simulink subsystem "Trot_planning"  (R2022b)
settings: Solver=VariableStepAuto  StartTime=0.0  StopTime=10.0  RelTol=1e-3
undefined symbols (not defined in the file or in its folder): D, DiscIntNeverNeededParam, P
settings Model: Creator=LiAn  LastModifiedBy=LiAn

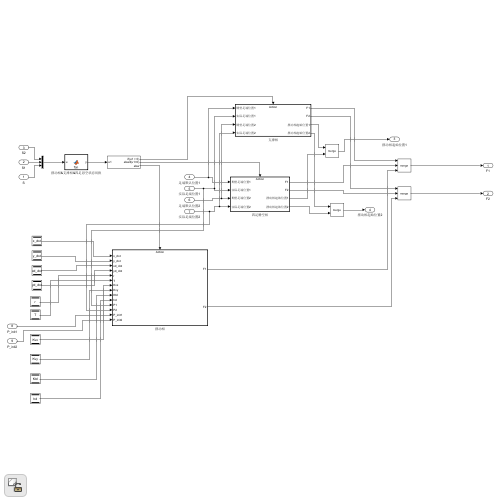
[thumbnail: Simulink's stored preview of the top-level diagram]
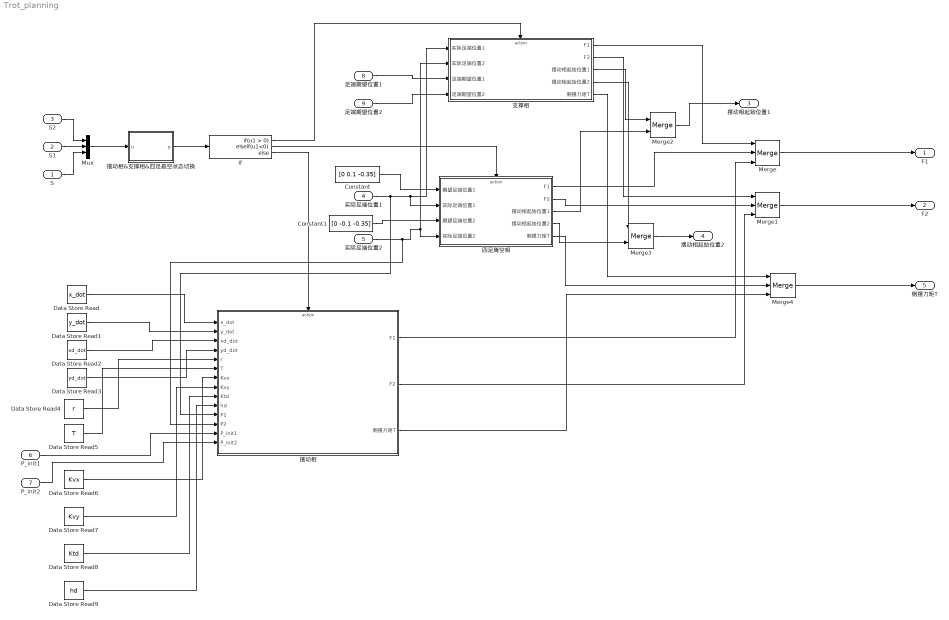
== system Trot_planning ==
  S : Inport
  S1 : Inport  Port=2
  S2 : Inport  Port=3
  实际足端位置1 : Inport  Port=4
  实际足端位置2 : Inport  Port=5
  P_init1 : Inport  Port=6
  P_init2 : Inport  Port=7
  足端期望位置1 : Inport  Port=8
  足端期望位置2 : Inport  Port=9
  Constant : Constant  Value=[0 0.1 -0.35]
  Constant1 : Constant  Value=[0 -0.1 -0.35]
  Data Store Read : DataStoreRead  DataStoreName=x_dot  IndexOptions=Index vector (dialog)  Indices=1  OutputSizes=1
  Data Store Read1 : DataStoreRead  DataStoreName=y_dot  IndexOptions=Index vector (dialog)  Indices=1  OutputSizes=1
  Data Store Read2 : DataStoreRead  DataStoreName=xd_dot  IndexOptions=Index vector (dialog)  Indices=1  OutputSizes=1
  Data Store Read3 : DataStoreRead  DataStoreName=yd_dot  IndexOptions=Index vector (dialog)  Indices=1  OutputSizes=1
  Data Store Read4 : DataStoreRead  DataStoreName=r  IndexOptions=Index vector (dialog)  Indices=1  OutputSizes=1
  Data Store Read5 : DataStoreRead  DataStoreName=T  IndexOptions=Index vector (dialog)  Indices=1  OutputSizes=1
  Data Store Read6 : DataStoreRead  DataStoreName=Kvx  IndexOptions=Index vector (dialog)  Indices=1  OutputSizes=1
  Data Store Read7 : DataStoreRead  DataStoreName=Kvy  IndexOptions=Index vector (dialog)  Indices=1  OutputSizes=1
  Data Store Read8 : DataStoreRead  DataStoreName=Ktd  IndexOptions=Index vector (dialog)  Indices=1  OutputSizes=1
  Data Store Read9 : DataStoreRead  DataStoreName=hd  IndexOptions=Index vector (dialog)  Indices=1  OutputSizes=1
  If : If  ElseIfExpressions=u1<0
  Merge : Merge  Inputs=3
  Merge1 : Merge  Inputs=3
  Merge2 : Merge
  Merge3 : Merge
  Merge4 : Merge  Inputs=3
  Mux : Mux  Inputs=3
  四足腾空相 : Subsystem  TreatAsAtomicUnit=on  mask{P=P, D=D}
      mask prompts: P "比例系数P"; D "阻尼系数D"
      mask DialogControl ParameterGroupVar Prompt: 参数
  摆动相 : Subsystem  TreatAsAtomicUnit=on
  摆动相&支撑相&四足悬空状态切换 : MATLAB Function  TreatAsAtomicUnit=on
  支撑相 : Subsystem  TreatAsAtomicUnit=on
  F1 : Outport
  F2 : Outport  Port=2
  摆动相起始位置1 : Outport  Port=3
  摆动相起始位置2 : Outport  Port=4
  侧摆力矩T : Outport  Port=5
  wires:
  S1/1 -> Mux/2
  S2/1 -> Mux/1
  S/1 -> Mux/3
  Mux/1 -> 摆动相&支撑相&四足悬空状态切换/1(u)
  摆动相&支撑相&四足悬空状态切换/1(y) -> If/1
  If/3 -> 摆动相/Action
  If/2 -> 四足腾空相/Action
  If/1 -> 支撑相/Action
  实际足端位置1/1 -> 四足腾空相/2(实际足端位置1), 支撑相/1(实际足端位置1), 摆动相/11(P1)
  实际足端位置2/1 -> 四足腾空相/4(实际足端位置2), 支撑相/2(实际足端位置2), 摆动相/12(P2)
  Merge/1 -> F1/1
  Merge1/1 -> F2/1
  四足腾空相/2(F2) -> Merge1/2
  四足腾空相/1(F1) -> Merge/2
  四足腾空相/4(摆动相起始位置2) -> Merge3/2
  四足腾空相/3(摆动相起始位置1) -> Merge2/2
  支撑相/1(F1) -> Merge/1
  支撑相/2(F2) -> Merge1/1
  支撑相/3(摆动相起始位置1) -> Merge2/1
  Merge2/1 -> 摆动相起始位置1/1
  支撑相/4(摆动相起始位置2) -> Merge3/1
  Merge3/1 -> 摆动相起始位置2/1
  Data Store Read/1 -> 摆动相/1(x_dot)
  Data Store Read1/1 -> 摆动相/2(y_dot)
  Data Store Read2/1 -> 摆动相/3(xd_dot)
  Data Store Read3/1 -> 摆动相/4(yd_dot)
  Data Store Read4/1 -> 摆动相/5(r)
  Data Store Read5/1 -> 摆动相/6(T)
  Data Store Read6/1 -> 摆动相/7(Kvx)
  Data Store Read7/1 -> 摆动相/8(Kvy)
  Data Store Read8/1 -> 摆动相/9(Ktd)
  Data Store Read9/1 -> 摆动相/10(hd)
  P_init1/1 -> 摆动相/13(P_init1)
  摆动相/1(F1) -> Merge/3
  摆动相/2(F2) -> Merge1/3
  P_init2/1 -> 摆动相/14(P_init2)
  Constant/1 -> 四足腾空相/1(期望足端位置1)
  Constant1/1 -> 四足腾空相/3(期望足端位置2)
  足端期望位置1/1 -> 支撑相/3(足端期望位置1)
  足端期望位置2/1 -> 支撑相/4(足端期望位置2)
  支撑相/5(侧摆力矩T) -> Merge4/1
  四足腾空相/5(侧摆力矩T) -> Merge4/2
  摆动相/3(侧摆力矩T) -> Merge4/3
  Merge4/1 -> 侧摆力矩T/1

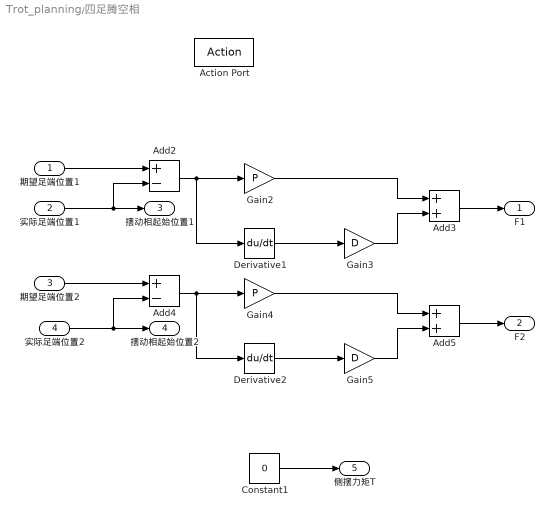
== system Trot_planning/四足腾空相 ==
  期望足端位置1 : Inport
  实际足端位置1 : Inport  Port=2
  期望足端位置2 : Inport  Port=3
  实际足端位置2 : Inport  Port=4
  Action Port : ActionPort
  Add2 : Sum  Inputs=+-
  Add3 : Sum
  Add4 : Sum  Inputs=+-
  Add5 : Sum
  Constant1 : Constant  Value=0
  Derivative1 : Derivative
  Derivative2 : Derivative
  Gain2 : Gain  Gain=P
  Gain3 : Gain  Gain=D
  Gain4 : Gain  Gain=P
  Gain5 : Gain  Gain=D
  F1 : Outport
  F2 : Outport  Port=2
  摆动相起始位置1 : Outport  Port=3
  摆动相起始位置2 : Outport  Port=4
  侧摆力矩T : Outport  Port=5
  wires:
  Constant1/1 -> 侧摆力矩T/1
  Add5/1 -> F2/1
  Gain5/1 -> Add5/2
  Add4/1 -> Gain4/1, Derivative2/1
  实际足端位置2/1 -> 摆动相起始位置2/1, Add4/2
  Gain4/1 -> Add5/1
  Derivative2/1 -> Gain5/1
  期望足端位置2/1 -> Add4/1
  期望足端位置1/1 -> Add2/1
  Derivative1/1 -> Gain3/1
  Gain2/1 -> Add3/1
  实际足端位置1/1 -> 摆动相起始位置1/1, Add2/2
  Add2/1 -> Derivative1/1, Gain2/1
  Gain3/1 -> Add3/2
  Add3/1 -> F1/1

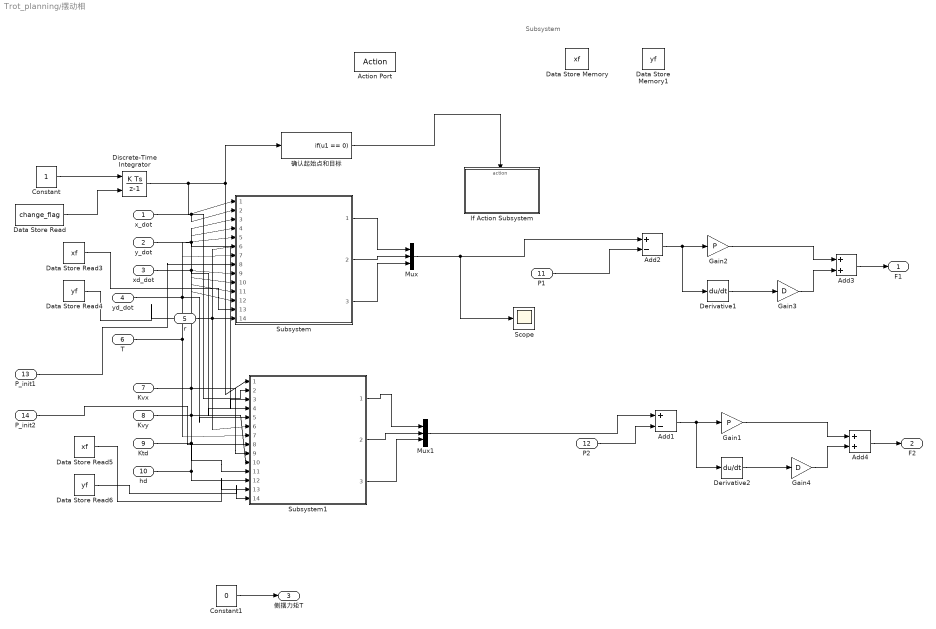
== system Trot_planning/摆动相 ==
  note: Subsystem
  x_dot : Inport
  y_dot : Inport  Port=2
  xd_dot : Inport  Port=3
  yd_dot : Inport  Port=4
  r : Inport  Port=5
  T : Inport  Port=6
  Kvx : Inport  Port=7
  Kvy : Inport  Port=8
  Ktd : Inport  Port=9
  hd : Inport  Port=10
  P1 : Inport  Port=11
  P2 : Inport  Port=12
  P_init1 : Inport  Port=13
  P_init2 : Inport  Port=14
  Action Port : ActionPort
  Add1 : Sum  Inputs=+-
  Add2 : Sum  Inputs=+-
  Add3 : Sum
  Add4 : Sum
  Constant : Constant
  Constant1 : Constant  Value=0
  Data Store Memory : DataStoreMemory  DataStoreName=xf  WriteAfterWriteMsg=warning  ShowAdditionalParam=off
  Data Store Memory1 : DataStoreMemory  DataStoreName=yf  WriteAfterWriteMsg=warning  ShowAdditionalParam=off
  Data Store Read : DataStoreRead  DataStoreName=change_flag  IndexOptions=Index vector (dialog)  Indices=1  OutputSizes=1
  Data Store Read3 : DataStoreRead  DataStoreName=xf  IndexOptions=Index vector (dialog)  Indices=1  OutputSizes=1
  Data Store Read4 : DataStoreRead  DataStoreName=yf  IndexOptions=Index vector (dialog)  Indices=1  OutputSizes=1
  Data Store Read5 : DataStoreRead  DataStoreName=xf  IndexOptions=Index vector (dialog)  Indices=1  OutputSizes=1
  Data Store Read6 : DataStoreRead  DataStoreName=yf  IndexOptions=Index vector (dialog)  Indices=1  OutputSizes=1
  Derivative1 : Derivative
  Derivative2 : Derivative
  Discrete-Time Integrator : DiscreteIntegrator  ExternalReset=rising  SampleTime=-1  ICPrevOutput=DiscIntNeverNeededParam  ICPrevScaledInput=DiscIntNeverNeededParam
  Gain1 : Gain  Gain=P
  Gain2 : Gain  Gain=P
  Gain3 : Gain  Gain=D
  Gain4 : Gain  Gain=D
  If Action Subsystem : Subsystem  TreatAsAtomicUnit=on
  Mux : Mux  Inputs=3
  Mux1 : Mux  Inputs=3
  Scope : Scope
  Subsystem : Subsystem  ReferencedSubsystem=swing_planning
  Subsystem1 : Subsystem  ReferencedSubsystem=swing_planning
  确认起始点和目标 : If  IfExpression=u1 == 0  ShowElse=off
  F1 : Outport
  F2 : Outport  Port=2
  侧摆力矩T : Outport  Port=3
  wires:
  Subsystem/3 -> Mux/3
  Data Store Read4/1 -> Subsystem/14
  Data Store Read3/1 -> Subsystem/13
  P_init1/1 -> Subsystem/8
  Subsystem/1 -> Mux/1
  Subsystem/2 -> Mux/2
  Data Store Read6/1 -> Subsystem1/14
  Data Store Read5/1 -> Subsystem1/13
  确认起始点和目标/1 -> If Action Subsystem/Action
  Constant1/1 -> 侧摆力矩T/1
  P_init2/1 -> Subsystem1/8
  Subsystem1/2 -> Mux1/2
  Subsystem1/1 -> Mux1/1
  Subsystem1/3 -> Mux1/3
  Mux1/1 -> Add1/1
  Gain1/1 -> Add4/1
  P2/1 -> Add1/2
  Add1/1 -> Gain1/1, Derivative2/1
  Gain4/1 -> Add4/2
  Add4/1 -> F2/1
  Derivative2/1 -> Gain4/1
  Derivative1/1 -> Gain3/1
  Add3/1 -> F1/1
  Gain3/1 -> Add3/2
  Add2/1 -> Derivative1/1, Gain2/1
  P1/1 -> Add2/2
  Gain2/1 -> Add3/1
  Mux/1 -> Add2/1, Scope/1
  x_dot/1 -> Subsystem/2, Subsystem1/2
  hd/1 -> Subsystem1/12, Subsystem/12
  y_dot/1 -> Subsystem/3, Subsystem1/3
  r/1 -> Subsystem/6, Subsystem1/6
  Ktd/1 -> Subsystem/11, Subsystem1/11
  xd_dot/1 -> Subsystem/4, Subsystem1/4
  Kvx/1 -> Subsystem/9, Subsystem1/9
  Kvy/1 -> Subsystem/10, Subsystem1/10
  yd_dot/1 -> Subsystem/5, Subsystem1/5
  T/1 -> Subsystem/7, Subsystem1/7
  Discrete-Time Integrator/1 -> 确认起始点和目标/1, Subsystem1/1, Subsystem/1
  Data Store Read/1 -> Discrete-Time Integrator/2
  Constant/1 -> Discrete-Time Integrator/1

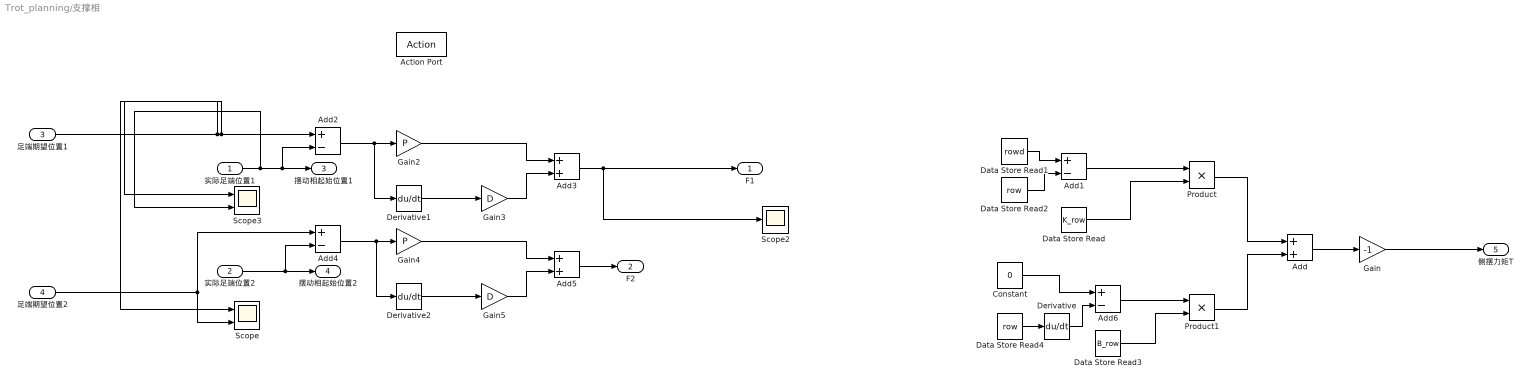
== system Trot_planning/支撑相 ==
  实际足端位置1 : Inport
  实际足端位置2 : Inport  Port=2
  足端期望位置1 : Inport  Port=3
  足端期望位置2 : Inport  Port=4
  Action Port : ActionPort
  Add : Sum
  Add{1..2,4,6} (4 alike) : Sum  Inputs=+-
  Add3 : Sum
  Add5 : Sum
  Constant : Constant  Value=0
  Data Store Read : DataStoreRead  DataStoreName=K_row  IndexOptions=Index vector (dialog)  Indices=1  OutputSizes=1
  Data Store Read1 : DataStoreRead  DataStoreName=rowd  IndexOptions=Index vector (dialog)  Indices=1  OutputSizes=1
  Data Store Read2 : DataStoreRead  DataStoreName=row  IndexOptions=Index vector (dialog)  Indices=1  OutputSizes=1
  Data Store Read3 : DataStoreRead  DataStoreName=B_row  IndexOptions=Index vector (dialog)  Indices=1  OutputSizes=1
  Data Store Read4 : DataStoreRead  DataStoreName=row  IndexOptions=Index vector (dialog)  Indices=1  OutputSizes=1
  Derivative : Derivative
  Derivative1 : Derivative
  Derivative2 : Derivative
  Gain : Gain  Gain=-1
  Gain2 : Gain  Gain=P
  Gain3 : Gain  Gain=D
  Gain4 : Gain  Gain=P
  Gain5 : Gain  Gain=D
  Product : Product
  Product1 : Product
  Scope : Scope  NumInputPorts=2
  Scope2 : Scope
  Scope3 : Scope  NumInputPorts=2
  F1 : Outport
  F2 : Outport  Port=2
  摆动相起始位置1 : Outport  Port=3
  摆动相起始位置2 : Outport  Port=4
  侧摆力矩T : Outport  Port=5
  wires:
  Gain/1 -> 侧摆力矩T/1
  Data Store Read3/1 -> Product1/2
  Data Store Read2/1 -> Add1/2
  Data Store Read/1 -> Product/2
  Derivative/1 -> Add6/2
  Data Store Read4/1 -> Derivative/1
  Constant/1 -> Add6/1
  Add1/1 -> Product/1
  Product1/1 -> Add/2
  Add/1 -> Gain/1
  Product/1 -> Add/1
  Data Store Read1/1 -> Add1/1
  Add6/1 -> Product1/1
  实际足端位置1/1 -> 摆动相起始位置1/1, Add2/2, Scope3/2
  Gain4/1 -> Add5/1
  Derivative2/1 -> Gain5/1
  实际足端位置2/1 -> 摆动相起始位置2/1, Add4/2
  Derivative1/1 -> Gain3/1
  足端期望位置2/1 -> Scope/2, Add4/1
  Add5/1 -> F2/1
  Add4/1 -> Gain4/1, Derivative2/1
  Gain5/1 -> Add5/2
  Add3/1 -> F1/1, Scope2/1
  Gain3/1 -> Add3/2
  Add2/1 -> Derivative1/1, Gain2/1
  Gain2/1 -> Add3/1
  足端期望位置1/1 -> Add2/1, Scope/1, Scope3/1

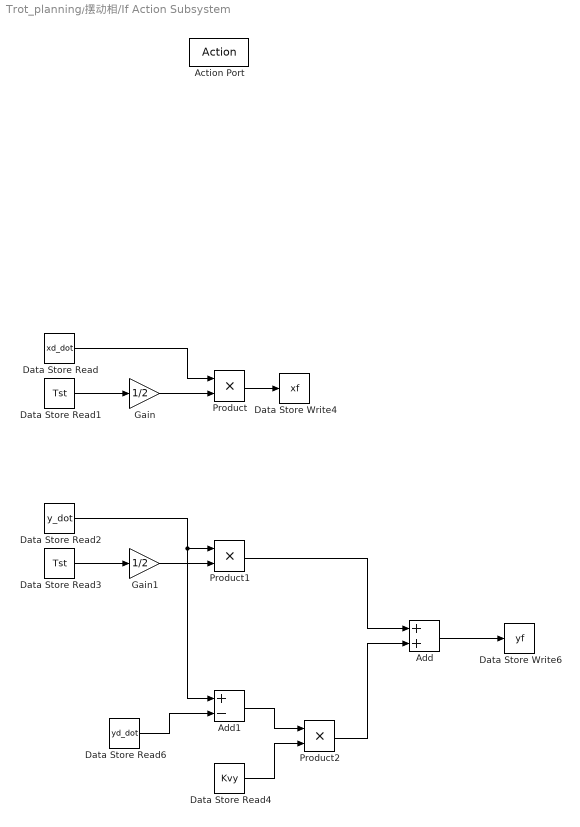
== system Trot_planning/摆动相/If Action Subsystem ==
  Action Port : ActionPort
  Add : Sum
  Add1 : Sum  Inputs=+-
  Data Store Read : DataStoreRead  DataStoreName=xd_dot  IndexOptions=Index vector (dialog)  Indices=1  OutputSizes=1
  Data Store Read1 : DataStoreRead  DataStoreName=Tst  IndexOptions=Index vector (dialog)  Indices=1  OutputSizes=1
  Data Store Read2 : DataStoreRead  DataStoreName=y_dot  IndexOptions=Index vector (dialog)  Indices=1  OutputSizes=1
  Data Store Read3 : DataStoreRead  DataStoreName=Tst  IndexOptions=Index vector (dialog)  Indices=1  OutputSizes=1
  Data Store Read4 : DataStoreRead  DataStoreName=Kvy  IndexOptions=Index vector (dialog)  Indices=1  OutputSizes=1
  Data Store Read6 : DataStoreRead  DataStoreName=yd_dot  IndexOptions=Index vector (dialog)  Indices=1  OutputSizes=1
  Data Store Write4 : DataStoreWrite  DataStoreName=xf  IndexOptions=Index vector (dialog)  Indices=1  OutputSizes=1
  Data Store Write6 : DataStoreWrite  DataStoreName=yf  IndexOptions=Index vector (dialog)  Indices=1  OutputSizes=1
  Gain : Gain  Gain=1/2
  Gain1 : Gain  Gain=1/2
  Product : Product
  Product1 : Product
  Product2 : Product
  wires:
  Add/1 -> Data Store Write6/1
  Product2/1 -> Add/2
  Data Store Read4/1 -> Product2/2
  Add1/1 -> Product2/1
  Data Store Read6/1 -> Add1/2
  Product1/1 -> Add/1
  Data Store Read2/1 -> Product1/1, Add1/1
  Gain1/1 -> Product1/2
  Data Store Read3/1 -> Gain1/1
  Product/1 -> Data Store Write4/1
  Data Store Read1/1 -> Gain/1
  Gain/1 -> Product/2
  Data Store Read/1 -> Product/1

== matlab function Trot_planning/摆动相&支撑相&四足悬空状态切换 ==
  data: u input; y output
function y = fcn(u)

if(u(3) == -1)
    y=-1;%四足腾空相
elseif(u(3)==u(1) || u(3)==u(2))
    y=0;%摆动相
else
    y=1;%支撑相
end
end
